simulink model "sysgenIIR"  (Simulink 7.2)
settings: Solver=ode45  StartTime=0.0  StopTime=10000  RelTol=1e-3
PreLoadFcn:
  | xlrequire('PreLoadFcn')
undefined symbols (not defined in the file or in its folder): num_channels
libraries: xbsIndex_r4 x128, xbsCopyrightNotice_r4 x1
settings Model: Creator=alexc  LastModifiedBy=juttu
settings DataIOCC: SignalLoggingName=sigsOut
settings OptimizationCC: BlockReduction=off  BooleanDataType=off  InlineInvariantSignals=on  InitFltsAndDblsToZero=on
settings DebuggingCC: SaveWithParameterizedLinksMsg=none  SignalResolutionControl=TryResolveAllWithWarning  SolverPrmCheckMsg=none  MultiTaskDSMMsg=warning  MultiTaskCondExecSysMsg=none  StrictBusMsg=None
settings HardwareCC: TargetUnknown=on
settings RTWCC: IncludeERTFirstTime=on
settings GRTTargetCC: TargetFcnLib=ansi_tfl_tmw.mat

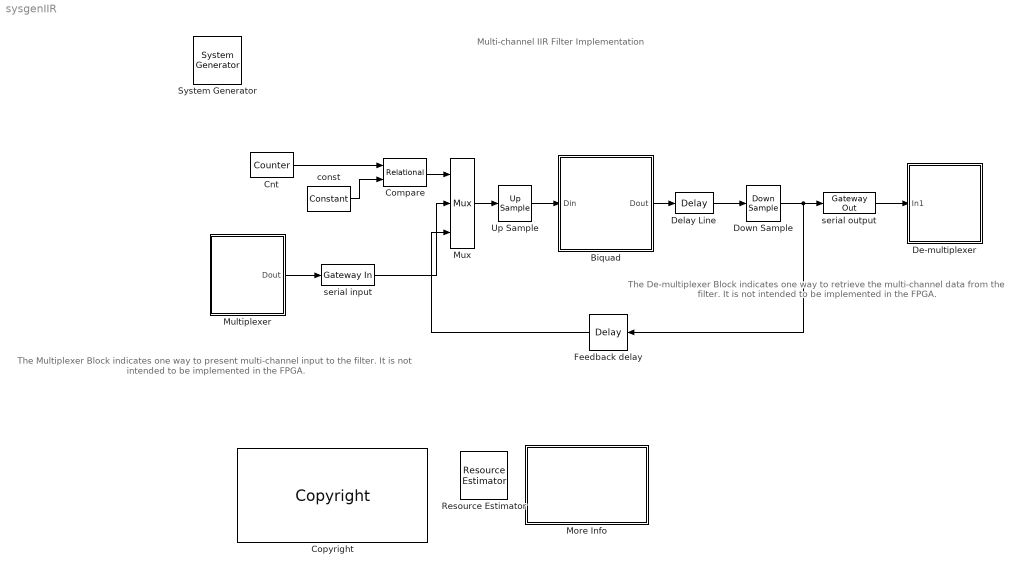
== system sysgenIIR ==
  note: Multi-channel IIR Filter Implementation
  note: The Multiplexer Block indicates one way to present
      | multi-channel input to the filter.  It is not intended to
      | be implemented in the FPGA.
  note: The De-multiplexer Block indicates one
      | way to retrieve the multi-channel data
      | from the filter. It is not intended to be
      | implemented in the FPGA.
  " System Generator" : xbsIndex_r4/ System Generator  Tag=genX  SystemSampleTime=-1  xilinxfamily=virtex5  part=xc5vsx50t  speed=-1  package=ff1136  synthesis_tool=XST  clock_wrapper=Clock Enables  directory=./netlist  testbench=on  simulink_period=1  sysclk_period=22  dcm_input_clock_period=100  incr_netlist=off  trim_vbits=Everywhere in SubSystem  dbl_ovrd=According to Block Masks  core_generation=According to Block Masks  run_coregen=off  deprecated_control=off  eval_field=0  block_type=sysgen
      settings: block_version=9.2.00
  Biquad : Subsystem
  Cnt : xbsIndex_r4/Counter  cnt_type=Count Limited  cnt_to=4*num_channels-1  operation=Up  start_count=0  cnt_by_val=1  arith_type=Unsigned  n_bits=ceil(log2(4*num_channels))  bin_pt=0  load_pin=off  rst=off  en=off  explicit_period=off  period=5  dbl_ovrd=off  use_behavioral_HDL=off  implementation=Fabric  use_rpm=off  block_type=counter
      settings: infoedit="Configurable up, down and up/down counter.<P><P>Hardware notes: Free running counters are the least expensive in hardware.  A count limited counter is implemented by combining a counter with a comparator."  xl_area=[4 6 0 8 0 0 0]  block_version=VER_STRING_GOES_HERE
  Compare : xbsIndex_r4/Relational  mode=a>b  en=off  latency=0  dbl_ovrd=off  block_type=relational
      settings: xl_area=[3 0 0 6 0 0 0]  block_version=VER_STRING_GOES_HERE
  Copyright : xbsCopyrightNotice_r4/Copyright  copyrighttext="Copyright (c) 2009  by  Xilinx, Inc. All rights reserved.<br><br>This file contains proprietary, confidential information of Xilinx, Inc., is distributed under licensefrom Xilinx, Inc., and may be used, copied and/or disclosed only pursuant to the terms of a valid licenseagreement with Xilinx, Inc. Xilinx hereby grants you a license to use this file solely for design,simulation, implementation and creation of design files limited to Xilinx devices or technologies. Use with non-Xilinx devices or technologies is expressly prohibited and immediately terminates your license unless covered by a separate agreement.<br><br>Xilinx is providing this design, code, or information \"as-is\" solely for use in developing programs and solutions for Xilinx devices, with no obligation on the part of Xilinx to provide support. By providingthis design, code, or information as one possible implementation of this feature, application or standard,Xilinx is making no representation that this implementation is free from any claims of infringement. Youare responsible for obtaining any rights you may require for your implementation. Xilinx expressly disclaimsany warranty whatsoever with respect to the adequacy of the implementation, including but not limited to anywarranties or representations that this implementation is free from claims of infringement, implied warrantiesof merchantability or fitness for a particular purpose.<br><br>Xilinx products are not intended for use in life support appliances, devices, or systems. Use in such applications is expressly prohibited.<br><br>Any modifications that are made to the Source Code are done at the user's sole risk and will be unsupported.<br><br>This copyright and support notice must be retained as part of this text at all times. (c) Copyright 1995-2009 Xilinx, Inc. All rights reserved."  block_type=copyright
      settings: block_version=10.1.00
      settings: infoedit=|
      | Copyright(C) 2008 by  Xilinx, Inc. All rights reserved.<br>
      | <br>
      | This file contains proprietary, confidential information of Xilinx, Inc., is distributed under license
      | from Xilinx, Inc., and may be used, copied and/or disclosed only pursuant to the terms of a valid license
      | agreement with Xilinx, Inc. Xilinx hereby grants you a license to use this file solely for design,
      | simulation, implementation and creation of design files limited to Xilinx devices or technologies. Use
      | with non-Xilinx devices or technologies is expressly prohibited and immediately terminates your license
      | unless covered by a separate agreement.<br>
      | <br>
      | Xilinx is providing this design, code, or information "as-is" solely for use in developing programs and
      | solutions for Xilinx devices, with no obligation on the part of Xilinx to provide support. By providing
      | this design, code, or information as one possible implementation of this feature, application or standard,
      | Xilinx is making no representation that this implementation is free from any claims of infringement. You
      | are responsible for obtaining any rights you may require for your implementation. Xilinx expressly disclaims
      | any warranty whatsoever with respect to the adequacy of the implementation, including but not limited to any
      | warranties or representations that this implementation is free from claims of infringement, implied warranties
      | of merchantability or fitness for a particular purpose.<br>
      | <br>
      | Xilinx products are not intended for use in life support appliances, devices, or systems. Use in such
      | applications is expressly prohibited.<br>
      | <br>
      | Any modifications that are made to the Source Code are done at the user's sole risk and will be unsupported.<br>
      | <br>
      | This copyright and support notice must be retained as part of this text at all times.
      | (c) Copyright 1995-2008 Xilinx, Inc. All rights reserved.
  De-multiplexer : Subsystem
  Delay Line : xbsIndex_r4/Delay  en=off  latency=3  dbl_ovrd=off  reg_retiming=off  block_type=delay
      settings: infoedit="Delay line having  configurable length.<P><P>Hardware notes: A delay line is a chain, each link of which is an SRL16 followed by a flip-flop. If register retiming is enabled, the delay line is a chain of flip-flops."  xl_area=[14 28 0 28 0 0 0]  block_version=VER_STRING_GOES_HERE
  Down Sample : xbsIndex_r4/Down Sample  sample_ratio=5  sample_phase=First Value of Frame  en=off  latency=0  dbl_ovrd=off  block_type=dsamp
      settings: xl_area=[29 29 0 28 0 0 0]  block_version=VER_STRING_GOES_HERE
  Feedback delay : xbsIndex_r4/Delay  Orientation=left  en=off  latency=14  dbl_ovrd=off  reg_retiming=off  block_type=delay
      settings: infoedit="Delay line having  configurable length.<P><P>Hardware notes: A delay line is a chain, each link of which is an SRL16 followed by a flip-flop. If register retiming is enabled, the delay line is a chain of flip-flops."  xl_area=[14 28 0 28 0 0 0]  block_version=VER_STRING_GOES_HERE
  More Info : Subsystem
      mask Display: disp('Double click\n for\n more information.')
  Multiplexer : Subsystem
  Mux : xbsIndex_r4/Mux  inputs=2  en=off  latency=0  precision=Full  arith_type="Signed  (2's comp)"  n_bits=8  bin_pt=2  quantization=Truncate  overflow=Wrap  dbl_ovrd=off  block_type=mux
      settings: xl_area=[14 0 0 28 0 0 0]  block_version=VER_STRING_GOES_HERE
  Resource Estimator : xbsIndex_r4/Resource Estimator  Tag=resEstTag  Slices=351  FFs=219  BRAMs=7  LUTs=625  IOBs=56  EBMs=8  TBUFs=0  xl_use_estimator_area=off  est_options=Estimate  xl_estimator_area=[351 219 7 625 56 8 0]  mrp_directory=./sysgenIIR_work  simulink_period=1  block_type=resource_estimator
      settings: AttributesFormatString=Resource\nEstimator  block_version=9.2.00
  Up Sample : xbsIndex_r4/Up Sample  sample_ratio=5  copy_samples=off  dbl_ovrd=off  block_type=usamp
      settings: infoedit="Up samples input data.  Inserted values  can be zeros or copies of the most recent input sample.<P><P>Hardware notes: No hardware is needed if inserted values are copies of the input sample; otherwise, a mux and single bit flip-flop are used."  xl_area=[15 1 0 28 0 0 0]  block_version=VER_STRING_GOES_HERE
  const : xbsIndex_r4/Constant  arith_type=Unsigned  const=num_channels-1  n_bits=ceil(log2(4*num_channels))  bin_pt=0  explicit_period=off  period=1  equ=P=C  opselect=C  inp2=PCIN>>17  opr=+  inp1=P  carry=CIN  dbl_ovrd=off  block_type=constant
      settings: block_version=VER_STRING_GOES_HERE
  serial input : xbsIndex_r4/Gateway In  arith_type="Signed  (2's comp)"  n_bits=data_width_nbits  bin_pt=data_width_frac  quantization="Round  (unbiased: +/- Inf)"  overflow=Saturate  period=5  dbl_ovrd=off  timing_constraint=Data Rate  locs_specified=off  LOCs={}  block_type=gatewayin
      settings: infoedit="Gateway in block.  Converts inputs of type Simulink integer, double and fixed point to  Xilinx fixed point type.<P><P>Hardware notes:  In hardware these blocks become top level input ports."  xl_area=[0 0 0 0 28 0 0]  block_version=VER_STRING_GOES_HERE
  serial output : xbsIndex_r4/Gateway Out  hdl_port=on  timing_constraint=Data Rate  locs_specified=off  LOCs={}  block_type=gatewayout
      settings: infoedit="Gateway out block.  Converts Xilinx fixed point inputs into ouputs of type Simulink integer, double, or fixed point.<P><P>Hardware notes:  In hardware these blocks become top level output ports or are discarded, depending on how they are configured."  xl_area=[0 0 0 0 28 0 0]  block_version=VER_STRING_GOES_HERE
  wires:
  Biquad/1(Dout) -> Delay Line/1
  Mux/1 -> Up Sample/1
  Feedback delay/1 -> Mux/3
  Up Sample/1 -> Biquad/1(Din)
  Down Sample/1 -> Feedback delay/1, serial output/1
  serial output/1 -> De-multiplexer/1(In1)
  serial input/1 -> Mux/2
  Compare/1 -> Mux/1
  Cnt/1 -> Compare/1
  const/1 -> Compare/2
  Multiplexer/1(Dout) -> serial input/1
  Delay Line/1 -> Down Sample/1

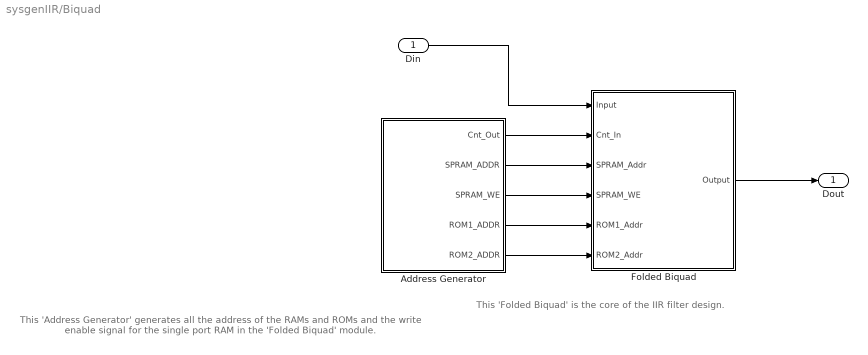
== system sysgenIIR/Biquad ==
  note: This 'Address Generator' generates all the address of the
      | RAMs and ROMs and the write enable signal for the single
      | port RAM in the 'Folded Biquad' module.
  note: This 'Folded Biquad' is the core of the IIR filter design.
  Din : Inport  OutDataType=sfix(16)  OutScaling=2^0
  Address Generator : Subsystem
  Folded Biquad : Subsystem
  Dout : Outport  OutDataType=sfix(16)  OutScaling=2^0
  wires:
  Address Generator/1(Cnt_Out) -> Folded Biquad/2(Cnt_In)
  Address Generator/2(SPRAM_ADDR) -> Folded Biquad/3(SPRAM_Addr)
  Address Generator/3(SPRAM_WE) -> Folded Biquad/4(SPRAM_WE)
  Address Generator/4(ROM1_ADDR) -> Folded Biquad/5(ROM1_Addr)
  Address Generator/5(ROM2_ADDR) -> Folded Biquad/6(ROM2_Addr)
  Folded Biquad/1(Output) -> Dout/1
  Din/1 -> Folded Biquad/1(Input)

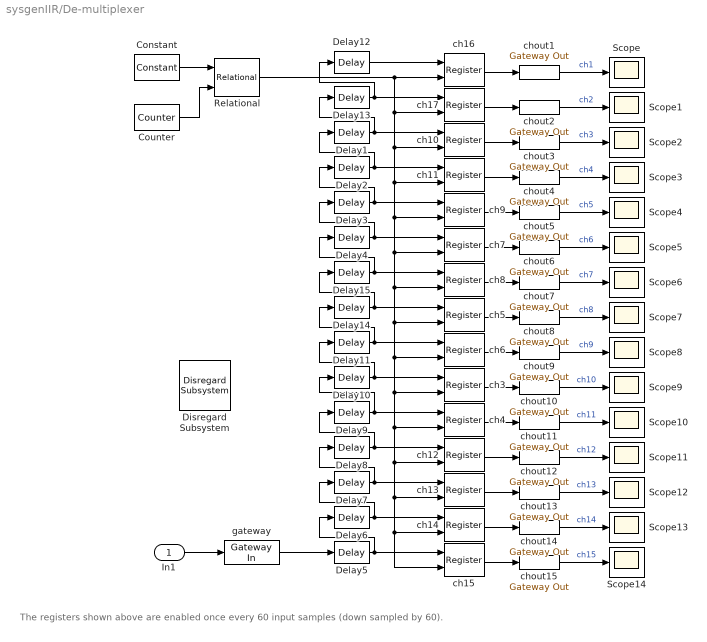
== system sysgenIIR/De-multiplexer ==
  note: The registers shown above are enabled once every 60 input samples (down sampled by 60).
  In1 : Inport  OutDataType=sfix(16)  OutScaling=2^0
  Constant : xbsIndex_r4/Constant  arith_type=Unsigned  const=0  n_bits=1  bin_pt=0  explicit_period=off  period=1  equ=P=C  opselect=C  inp2=PCIN>>17  opr=+  inp1=P  carry=CIN  dbl_ovrd=off  block_type=constant
      settings: block_version=VER_STRING_GOES_HERE
  Counter : xbsIndex_r4/Counter  cnt_type=Count Limited  cnt_to=4*num_channels-1  operation=Up  start_count=0  cnt_by_val=1  arith_type=Unsigned  n_bits=ceil(log2(4*num_channels))  bin_pt=0  load_pin=off  rst=off  en=off  explicit_period=off  period=5  dbl_ovrd=off  use_behavioral_HDL=off  use_rpm=off  implementation=Fabric  block_type=counter
      settings: infoedit="Configurable up, down and up/down counter.<P><P>Hardware notes: Free running counters are the least expensive in hardware.  A count limited counter is implemented by combining a counter with a comparator."  xl_area=[0, 0, 0, 0, 0, 0, 0]  block_version=VER_STRING_GOES_HERE
  Delay{1..15} (15 alike) : xbsIndex_r4/Delay  en=off  latency=1  dbl_ovrd=off  reg_retiming=off  block_type=delay
      settings: infoedit="Delay line having  configurable length.<P><P>Hardware notes: A delay line is a chain, each link of which is an SRL16 followed by a flip-flop. If register retiming is enabled, the delay line is a chain of flip-flops."  xl_area=[0, 0, 0, 0, 0, 0, 0]  block_version=VER_STRING_GOES_HERE
  Disregard Subsystem : xbsIndex_r4/Disregard Subsystem  Tag=discardX  block_type=disregard
      settings: infoedit="Place this block into any subsystem of a model to indicate that you do not wish System Generator to generate any hardware components for the subsystem.  This block can be used in combination with the Simulation Multiplexer block to build alternative simulation models for a portion of a design (e.g. to provide a simulation model for a black box)."  block_version=VER_STRING_GOES_HERE
  Relational : xbsIndex_r4/Relational  mode=a=b  en=off  latency=0  dbl_ovrd=off  block_type=relational
      settings: xl_area=[0, 0, 0, 0, 0, 0, 0]  block_version=VER_STRING_GOES_HERE
  Scope{,1..14} (15 alike) : Scope
      Scope settings: YMin=-1  YMax=1
      Scope10 settings: SaveName=ScopeData10
      Scope11 settings: SaveName=ScopeData11
      Scope12 settings: SaveName=ScopeData12
      Scope13 settings: YMin=0.425  YMax=0.65  SaveName=ScopeData13
      Scope14 settings: YMin=0.39  YMax=0.51  SaveName=ScopeData14
      Scope2 settings: SaveName=ScopeData2
      Scope3 settings: SaveName=ScopeData3
      Scope4 settings: SaveName=ScopeData4
      Scope5 settings: SaveName=ScopeData5
      Scope6 settings: SaveName=ScopeData6
      Scope7 settings: SaveName=ScopeData7
      Scope8 settings: SaveName=ScopeData8
      Scope9 settings: SaveName=ScopeData9
  ch{3..17} (15 alike) : xbsIndex_r4/Register  init=0  rst=off  en=on  dbl_ovrd=off  block_type=register
      settings: xl_area=[0, 0, 0, 0, 0, 0, 0]  block_version=VER_STRING_GOES_HERE
  chout{1..15} (15 alike) : xbsIndex_r4/Gateway Out  hdl_port=off  timing_constraint=Data Rate  locs_specified=off  LOCs={}  block_type=gatewayout
      settings: infoedit="Gateway out block.  Converts Xilinx fixed point inputs into ouputs of type Simulink integer, double, or fixed point.<P><P>Hardware notes:  In hardware these blocks become top level output ports or are discarded, depending on how they are configured."  xl_area=[0, 0, 0, 0, 0, 0, 0]  block_version=VER_STRING_GOES_HERE
  gateway : xbsIndex_r4/Gateway In  arith_type="Signed  (2's comp)"  n_bits=data_width_nbits  bin_pt=data_width_frac  quantization="Round  (unbiased: +/- Inf)"  overflow=Saturate  period=5  dbl_ovrd=off  timing_constraint=Data Rate  locs_specified=off  LOCs={}  block_type=gatewayin
      settings: infoedit="Gateway in block.  Converts inputs of type Simulink integer, double and fixed point to  Xilinx fixed point type.<P><P>Hardware notes:  In hardware these blocks become top level input ports."  xl_area=[0, 0, 0, 0, 0, 0, 0]  block_version=VER_STRING_GOES_HERE
  wires:
  Counter/1 -> Relational/2
  Constant/1 -> Relational/1
  gateway/1 -> Delay5/1
  Delay4/1 -> ch7/1, Delay3/1
  Delay3/1 -> ch9/1, Delay2/1
  Delay2/1 -> ch11/1, Delay1/1
  Delay1/1 -> ch10/1, Delay13/1
  Delay13/1 -> ch17/1, Delay12/1
  Delay12/1 -> ch16/1
  ch16/1 -> chout1/1
  chout1/1 -> Scope/1  "ch1"
  ch17/1 -> chout2/1
  chout2/1 -> Scope1/1  "ch2"
  ch10/1 -> chout3/1
  chout3/1 -> Scope2/1  "ch3"
  ch11/1 -> chout4/1
  chout4/1 -> Scope3/1  "ch4"
  ch9/1 -> chout5/1
  chout5/1 -> Scope4/1  "ch5"
  ch7/1 -> chout6/1
  chout6/1 -> Scope5/1  "ch6"
  chout7/1 -> Scope6/1  "ch7"
  ch8/1 -> chout7/1
  chout8/1 -> Scope7/1  "ch8"
  ch5/1 -> chout8/1
  chout9/1 -> Scope8/1  "ch9"
  ch6/1 -> chout9/1
  chout10/1 -> Scope9/1  "ch10"
  ch3/1 -> chout10/1
  chout11/1 -> Scope10/1  "ch11"
  ch4/1 -> chout11/1
  chout12/1 -> Scope11/1  "ch12"
  ch12/1 -> chout12/1
  chout13/1 -> Scope12/1  "ch13"
  ch13/1 -> chout13/1
  chout14/1 -> Scope13/1  "ch14"
  ch14/1 -> chout14/1
  chout15/1 -> Scope14/1  "ch15"
  ch15/1 -> chout15/1
  In1/1 -> gateway/1
  Relational/1 -> ch15/2, ch14/2, ch13/2, ch12/2, ch4/2, ch3/2, ch6/2, ch5/2, ch8/2, ch7/2, ch9/2, ch11/2, ch10/2, ch17/2, ch16/2
  Delay5/1 -> ch15/1, Delay6/1
  Delay6/1 -> ch14/1, Delay7/1
  Delay7/1 -> ch13/1, Delay8/1
  Delay8/1 -> ch12/1, Delay9/1
  Delay9/1 -> ch4/1, Delay10/1
  Delay10/1 -> ch3/1, Delay11/1
  Delay11/1 -> ch6/1, Delay14/1
  Delay14/1 -> ch5/1, Delay15/1
  Delay15/1 -> ch8/1, Delay4/1

== system sysgenIIR/More Info ==
  note: This design demonstrates how multiple IIR filters can be implemented using a single time-shared second-order section (biquad).  Specifically,
      | 15 distinct IIR filters, each consisting of four cascaded biquads, are realized in a "folded" architecture that uses a single hardware biquad.
      | Hardware folding is a technique to time-multiplex many algorithm operations onto a single functional unit (e.g. adder, multiplier).   For low
      | sample rate applications like audio and control, the required silicon area can be much reduced by time-sharing the hardware resources.
      |
      | In this design, the several individual folding techniques are employed:
      |  - the biquad is time-multiplexed among fifteen channels
      |  - the biquad is time-multiplexed among four cascade stages for each channel
      |  - the biquad is implemented using two multipliers and a single adder instead of the straightforward 5 multipliers and 4 adders (a biquad output
      |    is calculated in every 5 system clock cycles).
      |
      | The operating clock frequency for the top-level design as shown is approximately 66 MHz.  The speed for each channel (4-cascade-stage
      | IIR filter) is 50 MHz / (15 channels*4 biquads/channel*5 clks/biquad) = 220 KHz.
      |
      | This design occupies 379 Slice LUTs, 211Slice Registers, 423 Slice LUT-Flip Flop pairs, 4 Block RAMs, and 8  dedicated multipliers
      | of an xc5vsx50t-1 part (10.1.3 software, VHDL synthesized with XST).
  note: Multi-channel IIR Filter Implementation

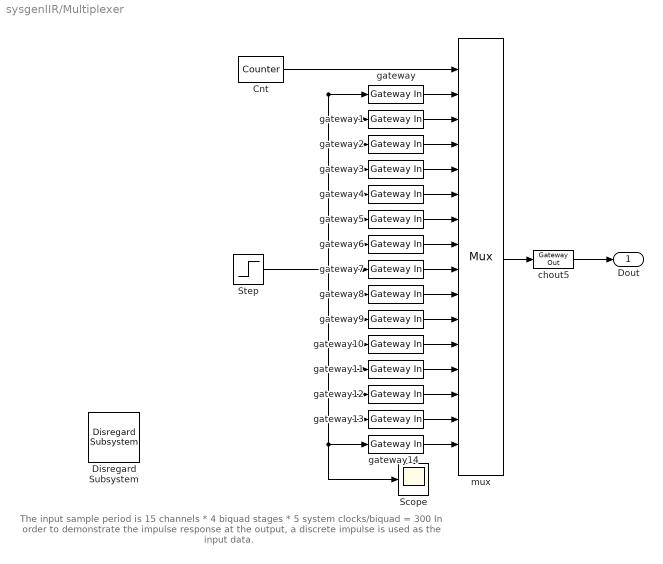
== system sysgenIIR/Multiplexer ==
  note: The input sample period is 15 channels * 4 biquad stages * 5 system clocks/biquad = 300
      | In order to demonstrate the impulse response at the output, a discrete impulse is used as
      | the input data.
  Cnt : xbsIndex_r4/Counter  cnt_type=Count Limited  cnt_to=num_channels-1  operation=Up  start_count=0  cnt_by_val=1  arith_type=Unsigned  n_bits=ceil(log2(num_channels))  bin_pt=0  load_pin=off  rst=off  en=off  explicit_period=off  period=5  dbl_ovrd=off  use_behavioral_HDL=off  use_rpm=off  implementation=Fabric  block_type=counter
      settings: infoedit="Configurable up, down and up/down counter.<P><P>Hardware notes: Free running counters are the least expensive in hardware.  A count limited counter is implemented by combining a counter with a comparator."  xl_area=[0, 0, 0, 0, 0, 0, 0]  block_version=VER_STRING_GOES_HERE
  Disregard Subsystem : xbsIndex_r4/Disregard Subsystem  Tag=discardX  block_type=disregard
      settings: infoedit="Place this block into any subsystem of a model to indicate that you do not wish System Generator to generate any hardware components for the subsystem.  This block can be used in combination with the Simulation Multiplexer block to build alternative simulation models for a portion of a design (e.g. to provide a simulation model for a black box)."  block_version=VER_STRING_GOES_HERE
  Scope : Scope
      settings: SaveName=ScopeData15
  Step : Step  Time=300  Before=1  After=0  SampleTime=5
  chout5 : xbsIndex_r4/Gateway Out  hdl_port=off  timing_constraint=Data Rate  locs_specified=off  LOCs={}  block_type=gatewayout
      settings: infoedit="Gateway out block.  Converts Xilinx fixed point inputs into ouputs of type Simulink integer, double, or fixed point.<P><P>Hardware notes:  In hardware these blocks become top level output ports or are discarded, depending on how they are configured."  xl_area=[0, 0, 0, 0, 0, 0, 0]  block_version=VER_STRING_GOES_HERE
  gateway{,1..14} (15 alike) : xbsIndex_r4/Gateway In  arith_type="Signed  (2's comp)"  n_bits=data_width_nbits  bin_pt=data_width_frac  quantization="Round  (unbiased: +/- Inf)"  overflow=Saturate  period=5  dbl_ovrd=off  timing_constraint=Data Rate  locs_specified=off  LOCs={}  block_type=gatewayin
      settings: infoedit="Gateway in block.  Converts inputs of type Simulink integer, double and fixed point to  Xilinx fixed point type.<P><P>Hardware notes:  In hardware these blocks become top level input ports."  xl_area=[0, 0, 0, 0, 0, 0, 0]  block_version=VER_STRING_GOES_HERE
  mux : xbsIndex_r4/Mux  inputs=15  en=off  latency=0  precision=Full  arith_type="Signed  (2's comp)"  n_bits=8  bin_pt=2  quantization=Truncate  overflow=Wrap  dbl_ovrd=off  block_type=mux
      settings: xl_area=[0, 0, 0, 0, 0, 0, 0]  block_version=VER_STRING_GOES_HERE
  Dout : Outport  OutDataType=sfix(16)  OutScaling=2^0
  wires:
  mux/1 -> chout5/1
  chout5/1 -> Dout/1
  gateway/1 -> mux/2
  gateway1/1 -> mux/3
  gateway2/1 -> mux/4
  gateway3/1 -> mux/5
  gateway4/1 -> mux/6
  gateway5/1 -> mux/7
  gateway6/1 -> mux/8
  gateway7/1 -> mux/9
  gateway8/1 -> mux/10
  gateway9/1 -> mux/11
  gateway10/1 -> mux/12
  gateway11/1 -> mux/13
  gateway12/1 -> mux/14
  gateway13/1 -> mux/15
  gateway14/1 -> mux/16
  Step/1 -> gateway/1, gateway1/1, gateway3/1, gateway4/1, gateway6/1, gateway7/1, gateway8/1, gateway9/1, gateway10/1, gateway11/1, gateway12/1, gateway13/1, gateway14/1, Scope/1, gateway5/1, gateway2/1
  Cnt/1 -> mux/1

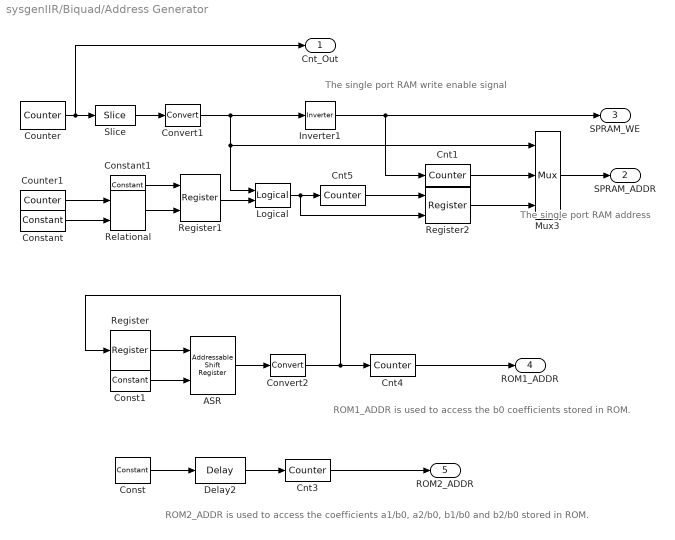
== system sysgenIIR/Biquad/Address Generator ==
  note: ROM1_ADDR is used to access
      | the b0 coefficients stored in ROM.
  note: ROM2_ADDR is used to access  the coefficients
      | a1/b0, a2/b0, b1/b0 and b2/b0 stored in ROM.
  note: The single port RAM address
  note: The single port RAM write enable signal
  ASR : xbsIndex_r4/Addressable Shift Register  infer_latency=on  depth=4  initVector=[0 0 0 0]  en=off  dbl_ovrd=off  use_behavioral_HDL=off  use_rpm=off  block_type=addrsr
      settings: infoedit="Delay of configurable length.  Any element in the delay line can be addressed and driven onto the output port.<P><P>Hardware notes: Implemented using SRL16s.  If a Virtex-II device is used, multiple SRLC16s are cascaded together."  xl_area=[1 0 0 1 0 0 0]  block_version=VER_STRING_GOES_HERE
  Cnt1 : xbsIndex_r4/Counter  cnt_type=Count Limited  cnt_to=16*num_channels-1  operation=Up  start_count=0  cnt_by_val=1  arith_type=Unsigned  n_bits=bits_needed_3  bin_pt=0  load_pin=off  rst=off  en=on  explicit_period=off  period=1  dbl_ovrd=off  use_behavioral_HDL=off  use_rpm=off  implementation=Fabric  block_type=counter
      settings: infoedit="Configurable up, down and up/down counter.<P><P>Hardware notes: Free running counters are the least expensive in hardware.  A count limited counter is implemented by combining a counter with a comparator."  xl_area=[6 8 0 11 0 0 0]  block_version=VER_STRING_GOES_HERE
  Cnt3 : xbsIndex_r4/Counter  cnt_type=Count Limited  cnt_to=20*num_channels-1  operation=Up  start_count=0  cnt_by_val=1  arith_type=Unsigned  n_bits=bits_needed_2  bin_pt=0  load_pin=off  rst=off  en=on  explicit_period=on  period=1  dbl_ovrd=off  use_behavioral_HDL=off  use_rpm=off  implementation=Fabric  block_type=counter
      settings: infoedit="Configurable up, down and up/down counter.<P><P>Hardware notes: Free running counters are the least expensive in hardware.  A count limited counter is implemented by combining a counter with a comparator."  xl_area=[7 9 0 12 0 0 0]  block_version=VER_STRING_GOES_HERE
  Cnt4 : xbsIndex_r4/Counter  cnt_type=Count Limited  cnt_to=4*num_channels-1  operation=Up  start_count=0  cnt_by_val=1  arith_type=Unsigned  n_bits=bits_needed_1  bin_pt=0  load_pin=off  rst=off  en=on  explicit_period=on  period=1  dbl_ovrd=off  use_behavioral_HDL=off  use_rpm=off  implementation=Fabric  block_type=counter
      settings: infoedit="Configurable up, down and up/down counter.<P><P>Hardware notes: Free running counters are the least expensive in hardware.  A count limited counter is implemented by combining a counter with a comparator."  xl_area=[4 6 0 8 0 0 0]  block_version=VER_STRING_GOES_HERE
  Cnt5 : xbsIndex_r4/Counter  cnt_type=Count Limited  cnt_to=16*num_channels-1  operation=Up  start_count=3  cnt_by_val=4  arith_type=Unsigned  n_bits=bits_needed_3  bin_pt=0  load_pin=off  rst=off  en=on  explicit_period=off  period=1  dbl_ovrd=off  use_behavioral_HDL=off  use_rpm=off  implementation=Fabric  block_type=counter
      settings: infoedit="Configurable up, down and up/down counter.<P><P>Hardware notes: Free running counters are the least expensive in hardware.  A count limited counter is implemented by combining a counter with a comparator."  xl_area=[6 8 0 11 0 0 0]  block_version=VER_STRING_GOES_HERE
  Const : xbsIndex_r4/Constant  arith_type=Boolean  const=1  n_bits=1  bin_pt=0  explicit_period=on  period=1  equ=P=C  opselect=C  inp2=PCIN>>17  opr=+  inp1=P  carry=CIN  dbl_ovrd=off  block_type=constant
      settings: block_version=VER_STRING_GOES_HERE
  Const1 : xbsIndex_r4/Constant  arith_type=Unsigned  const=3  n_bits=2  bin_pt=0  explicit_period=on  period=1  equ=P=C  opselect=C  inp2=PCIN>>17  opr=+  inp1=P  carry=CIN  dbl_ovrd=off  block_type=constant
      settings: block_version=VER_STRING_GOES_HERE
  Constant : xbsIndex_r4/Constant  arith_type=Unsigned  const=20*num_channels-7  n_bits=9  bin_pt=0  explicit_period=off  period=1  equ=P=C  opselect=C  inp2=PCIN>>17  opr=+  inp1=P  carry=CIN  dbl_ovrd=off  block_type=constant
      settings: block_version=VER_STRING_GOES_HERE
  Constant1 : xbsIndex_r4/Constant  arith_type=Boolean  const=1  n_bits=9  bin_pt=0  explicit_period=off  period=1  equ=P=C  opselect=C  inp2=PCIN>>17  opr=+  inp1=P  carry=CIN  dbl_ovrd=off  block_type=constant
      settings: block_version=VER_STRING_GOES_HERE
  Convert1 : xbsIndex_r4/Convert  arith_type=Boolean  n_bits=8  bin_pt=6  quantization=Truncate  overflow=Wrap  latency=0  dbl_ovrd=off  pipeline=off  block_type=convert
      settings: infoedit=The input is presented at the output after quantization and overflow effects.<P><P>Hardware notes: Additional hardware is used when rounding or saturation is selected and output width is less than the input width.  xl_area=[0 0 0 0 0 0 0]  block_version=VER_STRING_GOES_HERE
  Convert2 : xbsIndex_r4/Convert  arith_type=Boolean  n_bits=8  bin_pt=6  quantization=Truncate  overflow=Wrap  latency=0  dbl_ovrd=off  pipeline=off  block_type=convert
      settings: infoedit=The input is presented at the output after quantization and overflow effects.<P><P>Hardware notes: Additional hardware is used when rounding or saturation is selected and output width is less than the input width.  xl_area=[0 0 0 0 0 0 0]  block_version=VER_STRING_GOES_HERE
  Counter : xbsIndex_r4/Counter  cnt_type=Count Limited  cnt_to=4  operation=Up  start_count=0  cnt_by_val=1  arith_type=Unsigned  n_bits=3  bin_pt=0  load_pin=off  rst=off  en=off  explicit_period=off  period=1  dbl_ovrd=off  use_behavioral_HDL=off  use_rpm=off  implementation=Fabric  block_type=counter
      settings: infoedit="Configurable up, down and up/down counter.<P><P>Hardware notes: Free running counters are the least expensive in hardware.  A count limited counter is implemented by combining a counter with a comparator."  xl_area=[3 3 0 4 0 0 0]  block_version=VER_STRING_GOES_HERE
  Counter1 : xbsIndex_r4/Counter  cnt_type=Free Running  cnt_to=4  operation=Up  start_count=0  cnt_by_val=1  arith_type=Unsigned  n_bits=9  bin_pt=0  load_pin=off  rst=off  en=off  explicit_period=off  period=1  dbl_ovrd=off  use_behavioral_HDL=off  use_rpm=off  implementation=Fabric  block_type=counter
      settings: infoedit="Configurable up, down and up/down counter.<P><P>Hardware notes: Free running counters are the least expensive in hardware.  A count limited counter is implemented by combining a counter with a comparator."  xl_area=[5 9 0 9 0 0 0]  block_version=VER_STRING_GOES_HERE
  Delay2 : xbsIndex_r4/Delay  en=off  latency=20*num_channels-1  dbl_ovrd=off  reg_retiming=off  block_type=delay
      settings: infoedit="Delay line having  configurable length.<P><P>Hardware notes: A delay line is a chain, each link of which is an SRL16 followed by a flip-flop. If register retiming is enabled, the delay line is a chain of flip-flops."  xl_area=[18 18 0 18 0 0 0]  block_version=VER_STRING_GOES_HERE
  Inverter1 : xbsIndex_r4/Inverter  en=off  latency=0  dbl_ovrd=off  block_type=inv
      settings: xl_area=[1 0 0 1 0 0 0]  block_version=VER_STRING_GOES_HERE
  Logical : xbsIndex_r4/Logical  logical_function=AND  inputs=2  en=off  latency=0  precision=Full  arith_type=Unsigned  n_bits=8  bin_pt=2  align_bp=on  dbl_ovrd=off  block_type=logical
      settings: xl_area=[1 0 0 1 0 0 0]  block_version=VER_STRING_GOES_HERE
  Mux3 : xbsIndex_r4/Mux  inputs=2  en=off  latency=0  precision=User Defined  arith_type=Unsigned  n_bits=bits_needed_3  bin_pt=0  quantization=Truncate  overflow=Flag as error  dbl_ovrd=off  block_type=mux
      settings: xl_area=[4 0 0 8 0 0 0]  block_version=VER_STRING_GOES_HERE
  Register : xbsIndex_r4/Register  init=1  rst=off  en=off  dbl_ovrd=off  block_type=register
      settings: xl_area=[1 1 0 0 0 0 0]  block_version=VER_STRING_GOES_HERE
  Register1 : xbsIndex_r4/Register  init=0  rst=off  en=on  dbl_ovrd=off  block_type=register
      settings: xl_area=[1 1 0 0 0 0 0]  block_version=VER_STRING_GOES_HERE
  Register2 : xbsIndex_r4/Register  init=0  rst=off  en=on  dbl_ovrd=off  block_type=register
      settings: xl_area=[4 8 0 0 0 0 0]  block_version=VER_STRING_GOES_HERE
  Relational : xbsIndex_r4/Relational  mode=a=b  en=off  latency=0  dbl_ovrd=off  block_type=relational
      settings: xl_area=[3 0 0 5 0 0 0]  block_version=VER_STRING_GOES_HERE
  Slice : xbsIndex_r4/Slice  nbits=1  boolean_output=off  mode=Upper Bit Location + Width  bit1=0  base1=MSB of Input  bit0=0  base0=LSB of Input  dbl_ovrd=off  block_type=slice
      settings: infoedit="Extracts a given range of bits from each input sample and presents it at the output.  The output type is ordinarily unsigned with binary point at zero, but can be Boolean when the slice is one bit wide.<P><P>Hardware notes: In hardware this block costs nothing."  block_version=VER_STRING_GOES_HERE
  Cnt_Out : Outport  OutDataType=sfix(16)  OutScaling=2^0
  SPRAM_ADDR : Outport  Port=2  OutDataType=sfix(16)  OutScaling=2^0
  SPRAM_WE : Outport  Port=3  OutDataType=sfix(16)  OutScaling=2^0
  ROM1_ADDR : Outport  Port=4  OutDataType=sfix(16)  OutScaling=2^0
  ROM2_ADDR : Outport  Port=5  OutDataType=sfix(16)  OutScaling=2^0
  wires:
  Delay2/1 -> Cnt3/1
  Cnt3/1 -> ROM2_ADDR/1
  Const/1 -> Delay2/1
  Convert2/1 -> Register/1, Cnt4/1
  ASR/1 -> Convert2/1
  Register/1 -> ASR/1
  Const1/1 -> ASR/2
  Cnt4/1 -> ROM1_ADDR/1
  Inverter1/1 -> SPRAM_WE/1, Cnt1/1
  Convert1/1 -> Mux3/1, Logical/1, Inverter1/1
  Slice/1 -> Convert1/1
  Counter/1 -> Cnt_Out/1, Slice/1
  Mux3/1 -> SPRAM_ADDR/1
  Cnt1/1 -> Mux3/2
  Counter1/1 -> Relational/1
  Constant/1 -> Relational/2
  Relational/1 -> Register1/2
  Constant1/1 -> Register1/1
  Register1/1 -> Logical/2
  Logical/1 -> Cnt5/1, Register2/2
  Cnt5/1 -> Register2/1
  Register2/1 -> Mux3/3

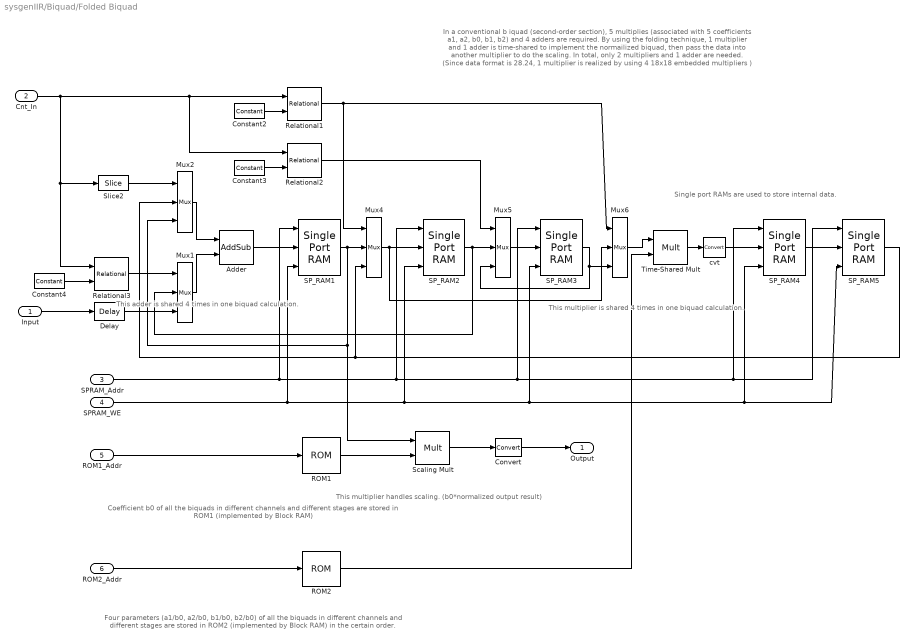
== system sysgenIIR/Biquad/Folded Biquad ==
  note: Coefficient b0 of all the biquads in
      | different channels and different stages
      | are stored in ROM1 (implemented by
      | Block RAM)
  note: Four parameters (a1/b0, a2/b0, b1/b0, b2/b0) of all the biquads in different
      | channels and different stages are stored in ROM2 (implemented by Block RAM)
      | in the certain order.
  note: In a conventional b   iquad (second-order section), 5 multiplies
      | (associated with 5 coefficients a1, a2, b0, b1, b2) and 4 adders
      | are required.  By using the folding technique, 1 multiplier and
      | 1 adder is time-shared to implement the normailized biquad,
      | then pass the data into another multiplier to do the scaling.
      | In total, only 2 multipliers and 1 adder are needed. (Since
      | data format is 28.24, 1 multiplier is realized by using
      | 4 18x18 embedded multipliers )
  note: This multiplier is
      | shared 4 times in
      | one biquad
      | calculation.
  note: This adder is
      | shared 4 times
      | in one biquad
      | calculation.
  note: Single port RAMs are used to store
      | internal data.
  note: This multiplier handles scaling.
      | (b0*normalized output result)
  Input : Inport  OutDataType=sfix(16)  OutScaling=2^0
  Cnt_In : Inport  Port=2  OutDataType=sfix(16)  OutScaling=2^0
  SPRAM_Addr : Inport  Port=3  OutDataType=sfix(16)  OutScaling=2^0
  SPRAM_WE : Inport  Port=4  OutDataType=sfix(16)  OutScaling=2^0
  ROM1_Addr : Inport  Port=5  OutDataType=sfix(16)  OutScaling=2^0
  ROM2_Addr : Inport  Port=6  OutDataType=sfix(16)  OutScaling=2^0
  Adder : xbsIndex_r4/AddSub  mode=Addition  use_carryin=off  use_carryout=off  en=off  latency=0  precision=User Defined  arith_type="Signed  (2's comp)"  n_bits=data_width_nbits  bin_pt=data_width_frac  quantization="Round  (unbiased: +/- Inf)"  overflow=Flag as error  dbl_ovrd=off  use_behavioral_HDL=on  pipelined=off  use_rpm=off  hw_selection=Fabric  block_type=addsub
      settings: xl_area=[15 0 0 28 0 0 0]  block_version=VER_STRING_GOES_HERE
  Constant2 : xbsIndex_r4/Constant  arith_type=Unsigned  const=0  n_bits=1  bin_pt=0  explicit_period=off  period=1  equ=P=C  opselect=C  inp2=PCIN>>17  opr=+  inp1=P  carry=CIN  dbl_ovrd=off  block_type=constant
      settings: block_version=VER_STRING_GOES_HERE
  Constant3 : xbsIndex_r4/Constant  arith_type=Unsigned  const=1  n_bits=1  bin_pt=0  explicit_period=off  period=1  equ=P=C  opselect=C  inp2=PCIN>>17  opr=+  inp1=P  carry=CIN  dbl_ovrd=off  block_type=constant
      settings: block_version=VER_STRING_GOES_HERE
  Constant4 : xbsIndex_r4/Constant  arith_type=Unsigned  const=3  n_bits=2  bin_pt=0  explicit_period=off  period=1  equ=P=C  opselect=C  inp2=PCIN>>17  opr=+  inp1=P  carry=CIN  dbl_ovrd=off  block_type=constant
      settings: block_version=VER_STRING_GOES_HERE
  Convert : xbsIndex_r4/Convert  arith_type="Signed  (2's comp)"  n_bits=data_width_nbits  bin_pt=data_width_frac  quantization=Truncate  overflow=Wrap  latency=0  dbl_ovrd=off  pipeline=off  block_type=convert
      settings: infoedit=The input is presented at the output after quantization and overflow effects.<P><P>Hardware notes: Additional hardware is used when rounding or saturation is selected and output width is less than the input width.  xl_area=[0 0 0 0 0 0 0]  block_version=VER_STRING_GOES_HERE
  Delay : xbsIndex_r4/Delay  en=off  latency=3  dbl_ovrd=off  reg_retiming=off  block_type=delay
      settings: infoedit="Delay line having  configurable length.<P><P>Hardware notes: A delay line is a chain, each link of which is an SRL16 followed by a flip-flop. If register retiming is enabled, the delay line is a chain of flip-flops."  xl_area=[14 28 0 28 0 0 0]  block_version=VER_STRING_GOES_HERE
  Mux{1..2,4..6} (5 alike) : xbsIndex_r4/Mux  inputs=2  en=off  latency=0  precision=User Defined  arith_type="Signed  (2's comp)"  n_bits=data_width_nbits  bin_pt=data_width_frac  quantization=Truncate  overflow=Flag as error  dbl_ovrd=off  block_type=mux
      settings: xl_area=[14 0 0 28 0 0 0]  block_version=VER_STRING_GOES_HERE
  ROM1 : xbsIndex_r4/ROM  depth=4*num_channels  initVector=coeff_b0  distributed_mem=Block RAM  rst=off  init_reg=0  en=off  latency=2  arith_type="Signed  (2's comp)"  n_bits=data_width_nbits  bin_pt=data_width_frac  dbl_ovrd=off  optimize=Area  use_rpm=off  block_type=sprom
      settings: xl_area=[0 28 1 0 0 0 0]  block_version=VER_STRING_GOES_HERE
  ROM2 : xbsIndex_r4/ROM  depth=20*num_channels  initVector=coeffs  distributed_mem=Block RAM  rst=off  init_reg=0  en=off  latency=1  arith_type="Signed  (2's comp)"  n_bits=data_width_nbits  bin_pt=data_width_frac  dbl_ovrd=off  optimize=Area  use_rpm=off  block_type=sprom
      settings: xl_area=[0 0 1 0 0 0 0]  block_version=VER_STRING_GOES_HERE
  Relational1 : xbsIndex_r4/Relational  mode=a!=b  en=off  latency=0  dbl_ovrd=off  block_type=relational
      settings: xl_area=[1 0 0 2 0 0 0]  block_version=VER_STRING_GOES_HERE
  Relational2 : xbsIndex_r4/Relational  mode=a!=b  en=off  latency=0  dbl_ovrd=off  block_type=relational
      settings: xl_area=[1 0 0 2 0 0 0]  block_version=VER_STRING_GOES_HERE
  Relational3 : xbsIndex_r4/Relational  mode=a=b  en=off  latency=0  dbl_ovrd=off  block_type=relational
      settings: xl_area=[1 0 0 2 0 0 0]  block_version=VER_STRING_GOES_HERE
  SP_RAM{1..5} (5 alike) : xbsIndex_r4/Single Port RAM  depth=16*num_channels  initVector=[zeros([1,16*num_channels])]  distributed_mem=Block RAM  write_mode=Read After Write  rst=off  init_reg=0  en=off  latency=1  dbl_ovrd=off  optimize=Area  use_rpm=off  block_type=spram
      settings: xl_area=[0 0 1 0 0 0 0]  block_version=8.2
  Scaling Mult : xbsIndex_r4/Mult  precision=User Defined  arith_type="Signed  (2's comp)"  n_bits=mult_width_nbits  bin_pt=mult_width_frac  quantization=Truncate  overflow=Flag as error  en=off  latency=0  dbl_ovrd=off  use_behavioral_HDL=off  use_embedded=on  opt=Speed  optimum_pipeline=off  pipeline=off  use_rpm=off  placement_style=Rectangular shape  block_type=mult
      settings: infoedit=Multiplies two values.<P><P>Hardware notes: To use the internal pipeline stage of the dedicated multiplier you must select 'Pipeline to Greatest Extent Possible'.  xl_area=[45 0 0 89 0 4 0]  block_version=VER_STRING_GOES_HERE
  Slice2 : xbsIndex_r4/Slice  nbits=1  boolean_output=off  mode=Lower Bit Location + Width  bit1=0  base1=MSB of Input  bit0=0  base0=LSB of Input  dbl_ovrd=off  block_type=slice
      settings: infoedit="Extracts a given range of bits from each input sample and presents it at the output.  The output type is ordinarily unsigned with binary point at zero, but can be Boolean when the slice is one bit wide.<P><P>Hardware notes: In hardware this block costs nothing."  block_version=VER_STRING_GOES_HERE
  Time-Shared Mult : xbsIndex_r4/Mult  precision=Full  arith_type="Signed  (2's comp)"  n_bits=mult_width_nbits  bin_pt=mult_width_frac  quantization=Truncate  overflow=Flag as error  en=off  latency=0  dbl_ovrd=off  use_behavioral_HDL=off  use_embedded=on  opt=Speed  optimum_pipeline=off  pipeline=off  use_rpm=off  placement_style=Rectangular shape  block_type=mult
      settings: infoedit=Multiplies two values.<P><P>Hardware notes: To use the internal pipeline stage of the dedicated multiplier you must select 'Pipeline to Greatest Extent Possible'.  xl_area=[46 0 0 91 0 4 0]  block_version=VER_STRING_GOES_HERE
  cvt : xbsIndex_r4/Convert  arith_type="Signed  (2's comp)"  n_bits=data_width_nbits  bin_pt=data_width_frac  quantization=Truncate  overflow=Wrap  latency=0  dbl_ovrd=off  pipeline=off  block_type=convert
      settings: infoedit=The input is presented at the output after quantization and overflow effects.<P><P>Hardware notes: Additional hardware is used when rounding or saturation is selected and output width is less than the input width.  xl_area=[0 0 0 0 0 0 0]  block_version=VER_STRING_GOES_HERE
  Output : Outport  OutDataType=sfix(16)  OutScaling=2^0
  wires:
  Time-Shared Mult/1 -> cvt/1
  Adder/1 -> SP_RAM1/2
  SP_RAM2/1 -> Mux5/2, Mux1/2
  Input/1 -> Delay/1
  Mux4/1 -> Mux6/2, SP_RAM2/2
  Mux5/1 -> SP_RAM3/2
  SP_RAM3/1 -> Mux6/3, Mux5/3
  cvt/1 -> SP_RAM4/2
  Delay/1 -> Mux1/3
  SP_RAM4/1 -> SP_RAM5/2
  Cnt_In/1 -> Relational1/1, Relational2/1, Relational3/1, Slice2/1
  SP_RAM1/1 -> Mux4/2, Mux2/3, Scaling Mult/1
  Constant2/1 -> Relational1/2
  Constant3/1 -> Relational2/2
  Relational2/1 -> Mux5/1
  Mux2/1 -> Adder/1
  Mux1/1 -> Adder/2
  Constant4/1 -> Relational3/2
  Relational3/1 -> Mux1/1
  Mux6/1 -> Time-Shared Mult/1
  SP_RAM5/1 -> Mux2/2, Mux4/3
  Slice2/1 -> Mux2/1
  ROM2/1 -> Time-Shared Mult/2
  Relational1/1 -> Mux4/1, Mux6/1
  Scaling Mult/1 -> Convert/1
  Convert/1 -> Output/1
  ROM1/1 -> Scaling Mult/2
  SPRAM_Addr/1 -> SP_RAM1/1, SP_RAM5/1, SP_RAM4/1, SP_RAM3/1, SP_RAM2/1
  SPRAM_WE/1 -> SP_RAM1/3, SP_RAM2/3, SP_RAM5/3, SP_RAM4/3, SP_RAM3/3
  ROM2_Addr/1 -> ROM2/1
  ROM1_Addr/1 -> ROM1/1
